simulink model "process_with_signal_with_filter_class576"  (Simulink 7.6)
settings: Solver=ode45  StartTime=0.0  StopTime=50  RelTol=1e-3
libraries: simulink x1
settings Model: Creator=administrator  LastModifiedBy=administrator

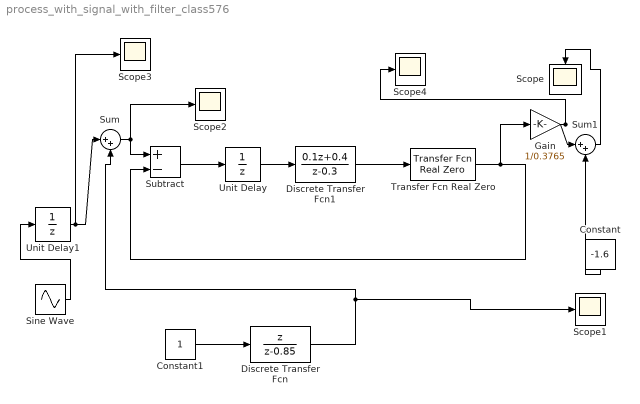
== system process_with_signal_with_filter_class576 ==
  Constant : Constant  Value=-1.6
  Constant1 : Constant
  Discrete Transfer Fcn : DiscreteTransferFcn  Numerator=[1 0]  Denominator=[1 -0.85]
  Discrete Transfer Fcn1 : DiscreteTransferFcn  Numerator=[0.1 0.4]  Denominator=[1 -0.3]
  Gain : Gain  Gain=1/0.3765
  Scope{,1..4} (5 alike) : Scope
      Scope1 settings: TimeRange=50  YMin=0  YMax=7
      Scope2 settings: TimeRange=50  YMin=-1  YMax=7  SaveName=ScopeData2
      Scope3 settings: SaveName=ScopeData3
      Scope4 settings: SaveName=ScopeData4
  Sine Wave : Sin  SampleTime=0
  Subtract : Sum  Inputs=+-
  Sum : Sum  Inputs=|++
  Sum1 : Sum  Inputs=|++
  Transfer Fcn Real Zero : simulink/Discrete/Transfer Fcn Real Zero  SystemSampleTime=-1  ZeroZ=0.85  ICPrevInput=0.0  DoSatur=off
  Unit Delay : UnitDelay
  Unit Delay1 : UnitDelay
  wires:
  Unit Delay/1 -> Discrete Transfer Fcn1/1
  Subtract/1 -> Unit Delay/1
  Sum/1 -> Subtract/1, Scope2/1
  Constant1/1 -> Discrete Transfer Fcn/1
  Discrete Transfer Fcn/1 -> Scope1/1, Sum/2
  Discrete Transfer Fcn1/1 -> Transfer Fcn Real Zero/1
  Transfer Fcn Real Zero/1 -> Gain/1, Subtract/2
  Constant/1 -> Sum1/2
  Sine Wave/1 -> Unit Delay1/1
  Unit Delay1/1 -> Scope3/1, Sum/1
  Sum1/1 -> Scope/1
  Gain/1 -> Scope4/1, Sum1/1
